simulink model "PID_loop_control"  (Simulink 3.00)
libraries: mathlib x4, execlib x1, reglib x1, arclib x1

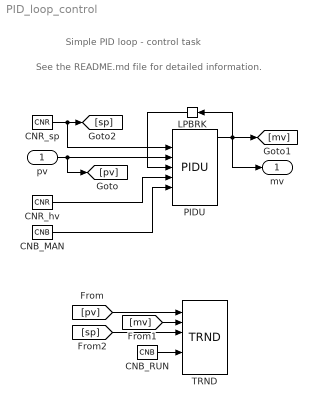
== system PID_loop_control ==
  note: See the README.md file for detailed information.
  note: Simple PID loop - control task
  pv : Inport  Port=1
  CNB_MAN : mathlib/CNB  YCN=off
  CNB_RUN : mathlib/CNB  YCN=on
  CNR_hv : mathlib/CNR  ycn=50
  CNR_sp : mathlib/CNR  ycn=22
  LPBRK : execlib/LPBRK  Orientation=left
  PIDU : reglib/PIDU  irtype=7: PID  RACT=off  k=4.9  ti=4.6  td=1.19  nd=2  b=0.65  c=0  tt=1  hilim=100  lolim=0  dz=0  icotype=1: Analog
  TRND : arclib/TRND  n=3  l=500  btype=8: Double  ptype1=1: Store  ptype2=1: Store  ptype3=1: Store  ptype4=1: Store  pfac=1  afac=0  arc=0  id=1  Title=Trend Title  timesrc=1
  mv : Outport  Port=1
  wires:
  CNB_MAN/1 -> PIDU/6
  CNB_RUN/1 -> TRND/5
  CNR_hv/1 -> PIDU/5
  CNR_sp/1 -> [sp], PIDU/2
  [pv] -> TRND/1
  [mv] -> TRND/2
  [sp] -> TRND/3
  LPBRK/1 -> PIDU/4
  PIDU/1 -> [mv], LPBRK/1, mv/1
  pv/1 -> [pv], PIDU/3
